simulink model "sfcndemo_cppcount"  (Simulink 7.6)
settings: Solver=FixedStepDiscrete  StartTime=0.0  StopTime=10  FixedStep=1  RelTol=1e-3
Description:
  | Bringing in C++ Code into a C++ S-function Including Code Generation Support
settings Model: Creator=The MathWorks Inc.  ExtModeTrigMode=oneshot  ExtModeArmWhenConnect=off  ExtModeAutoUpdateStatusClock=off
settings DataIOCC: LimitDataPoints=off  SaveOutput=off  SignalLogging=off  SaveTime=off  SignalLoggingName=logsOut
settings OptimizationCC: StateBitsets=on  DataBitsets=on  UseTempVars=on  InitFltsAndDblsToZero=on  BufferReusableBoundary=off
settings DebuggingCC: SaveWithParameterizedLinksMsg=none  SignalResolutionControl=TryResolveAllWithWarning  SolverPrmCheckMsg=none  MultiTaskDSMMsg=warning  MultiTaskCondExecSysMsg=none  SigSpecEnsureSampleTimeMsg=none
settings HardwareCC: ProdHWDeviceType=Specified  TargetHWDeviceType=32-bit Generic  ProdEqTarget=off
settings RTWCC: GenerateReport=on  RTWVerbose=off  ProcessScript=grt_make_rtw_hook  CustomSourceCode="#include \"sfun_cppcount_cpp.h\""  CustomInclude=../../../../simulink/src  CustomSource=sfun_cppcount_cpp.cpp  LaunchReport=on  TargetLang=C++  IncludeERTFirstTime=on
settings CodeAppCC: ForceParamTrailComments=on  CustomSymbolStrFcn=$F$N$M
settings GRTTargetCC: TargetFcnLib=ansi_tfl_tmw.mat

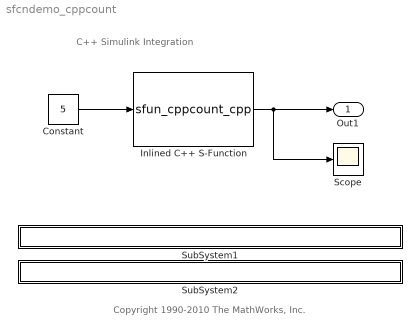
== system sfcndemo_cppcount ==
  note: C++ Simulink Integration
  note: Copyright 1990-2010 The MathWorks, Inc.
  Constant : Constant  Value=5
  Inlined C++ S-Function : S-Function  FunctionName=sfun_cppcount_cpp  EnableBusSupport=off
      mask Display: disp('Inlined C++\nS-Function');
  Scope : Scope
      settings: TimeRange=10  YMin=0  YMax=60
  SubSystem1 : Subsystem  mask{filename=sfun_cppcount_cpp.cpp}
      mask init:
      | x=sfundemo_maskdisp;
      settings: AttributesFormatString=\n  OpenFcn=sfundemo_openfcn
      mask Display: disp(x);
  SubSystem2 : Subsystem  mask{filename=sfun_cppcount_cpp.h}
      mask init:
      | x=sfundemo_maskdisp;
      settings: AttributesFormatString=\n  OpenFcn=sfundemo_openfcn
      mask Display: disp(x);
  Out1 : Outport
  wires:
  Inlined C++ S-Function/1 -> Out1/1, Scope/1
  Constant/1 -> Inlined C++ S-Function/1

== system sfcndemo_cppcount/SubSystem1 ==

== system sfcndemo_cppcount/SubSystem2 ==
